simulink model "B2_comparison_tool"  (R2021b)
settings: Solver=VariableStepAuto  StartTime=0.0  StopTime=10  RelTol=1e-3
values from neighbouring files (symbols this model uses):
  K_act = 50    [A10_simple_plant.m]    (also in A11_setup_script_pprz.m = 20; A1_setup_script.m = 20)
  K_act_inner = K_act*eye(4)    [A11_setup_script_pprz.m]    (also in A1_setup_script.m)
  K_ec_u = 1.5    [A11_setup_script_pprz.m]    (also in A1_setup_script.m = 5)
  K_ec_v = 1.5    [A11_setup_script_pprz.m]    (also in A1_setup_script.m = 5)
  K_ec_w = 1.5    [A11_setup_script_pprz.m]    (also in A1_setup_script.m = 5)
  K_u_d = 2.5    [A11_setup_script_pprz.m]    (also in A1_setup_script.m = 7)
  K_v_d = 2.5    [A11_setup_script_pprz.m]    (also in A1_setup_script.m = 7)
  K_w_d = 2.5    [A11_setup_script_pprz.m]    (also in A1_setup_script.m = 7)
  max_motor_rate = 30000    [A11_setup_script_pprz.m]    (also in A1_setup_script.m)
  max_omega_motor = 11000    [A11_setup_script_pprz.m]    (also in A1_setup_script.m)
  omega_c_motors = 50    [A11_setup_script_pprz.m]    (also in A1_setup_script.m)
  sampling_time = 1/frequency    (= 0.002)    [A11_setup_script_pprz.m]    (also in A12_sim_multi_run.m; A1_setup_script.m; A6_slow_actuator.m)
undefined symbols (not defined in the file or in its folder): K_ec_d_p, K_ec_d_q, K_ec_d_r, K_ec_dd_p, K_ec_dd_q, K_ec_dd_r, K_ec_p, K_ec_q, K_ec_r, K_p, K_p_d, K_p_dd, K_q, K_q_d, K_q_dd, K_r, K_r_d, K_r_dd
libraries: dspinverses x16, simulink_extras x8, aerolibutil x2, sharedutil x2, aerolibbdyn x2, aerolibatmos2 x2
(part 2 of 5)

== system B2_comparison_tool/System 0 - New/INDI w// RSPI ==
  " " : Constant  Value=[0;0;0;0]
  Constant : Constant  Value=0
  Constant1 : Constant  Value=max_omega_motor
  Constant2 : Constant  Value=max_motor_rate
  Constant3 : Constant  Value=sampling_time
  Constant4 : Constant  Value=2
  Constant5 : Constant  Value=0
  Demux : Demux
  Demux1 : Demux  Outputs=3
  Demux2 : Demux  Outputs=3
  ERROR CONTROLLER ATTITUDE : Subsystem
  ERROR CONTROLLER VELOCITY : Subsystem
  INTERNAL REFERENCE MODEL ATTITUDE : Subsystem
  INTERNAL REFERENCE MODEL VELOCITY : Subsystem
  MATLAB Function : MATLAB Function  TreatAsAtomicUnit=on
  Scope : Scope
  Scope1 : Scope
  Scope5 : Scope  NumInputPorts=3
  Scope6 : Scope  NumInputPorts=3
  Sum{9..10,14..17} (6 alike) : Sum  Inputs=|+-
  Sum{4..6,11..13} (6 alike) : Sum  Inputs=|++
  Vector Concatenate : Concatenate  NumInputs=6
  pqr_ref : Scope  NumInputPorts=3
  uvw_ref : Scope  NumInputPorts=3
  Motor_1_omega_input : Outport
  Motor_2_omega_input : Outport  Port=2
  Motor_3_omega_input : Outport  Port=3
  Motor_4_omega_input : Outport  Port=4
  wires:
  [Ixx] -> MATLAB Function/1(Ixx)
  [Iyy] -> MATLAB Function/2(Iyy)
  [Izz] -> MATLAB Function/3(Izz)
  [K_m] -> MATLAB Function/4(K_m)
  [K_t] -> MATLAB Function/5(K_t)
  [omega_1] -> MATLAB Function/6(Omega_1)
  [omega_2] -> MATLAB Function/7(Omega_2)
  [omega_3] -> MATLAB Function/8(Omega_3)
  [omega_4] -> MATLAB Function/9(Omega_4)
  [Phi] -> MATLAB Function/10(Phi)
  [Psi] -> MATLAB Function/11(Psi)
  [Theta] -> MATLAB Function/12(Theta)
  [m] -> MATLAB Function/15(m)
  Demux/1 -> Motor_1_omega_input/1
  Demux/2 -> Motor_2_omega_input/1
  Demux/3 -> Motor_3_omega_input/1
  Demux/4 -> Motor_4_omega_input/1
  [dv] -> MATLAB Function/16(dv)
  " "/1 -> MATLAB Function/17(desired_u)
  Constant1/1 -> MATLAB Function/18(max_omega_motor)
  Constant2/1 -> MATLAB Function/19(max_motor_rate)
  Constant3/1 -> MATLAB Function/20(sampling_time)
  MATLAB Function/1(u_out) -> Scope/1, Demux/1
  Constant4/1 -> MATLAB Function/21(max_iter)
  Constant/1 -> INTERNAL REFERENCE MODEL ATTITUDE/1(phi_cmd)
  Constant5/1 -> INTERNAL REFERENCE MODEL ATTITUDE/2(theta_cmd)
  INTERNAL REFERENCE MODEL VELOCITY/5(v_ref) -> ERROR CONTROLLER VELOCITY/2(v_ref), uvw_ref/2
  INTERNAL REFERENCE MODEL ATTITUDE/6(r_ref) -> ERROR CONTROLLER ATTITUDE/3(r_ref), pqr_ref/3
  Demux1/3 -> Sum14/2
  [u_des] -> INTERNAL REFERENCE MODEL VELOCITY/1(u_cmd)
  Sum9/1 -> Vector Concatenate/1
  ERROR CONTROLLER VELOCITY/1(ud_ec) -> Scope6/1, Sum5/2
  [yaw_des] -> INTERNAL REFERENCE MODEL ATTITUDE/3(psi_cmd)
  Vector Concatenate/1 -> Scope1/1, [dv]
  INTERNAL REFERENCE MODEL ATTITUDE/3(rd_ref) -> Sum13/1
  Demux1/1 -> Sum9/2
  INTERNAL REFERENCE MODEL ATTITUDE/5(q_ref) -> ERROR CONTROLLER ATTITUDE/2(q_ref), pqr_ref/2
  Demux2/3 -> Sum17/2
  Sum16/1 -> Vector Concatenate/5
  [pqr_dot_body] -> Demux1/1
  [AxAyAz_earth] -> Demux2/1
  Sum12/1 -> Sum17/1
  Sum10/1 -> Vector Concatenate/2
  Sum14/1 -> Vector Concatenate/3
  ERROR CONTROLLER ATTITUDE/2(qd_ec) -> Scope5/2, Sum11/2
  Demux2/2 -> Sum16/2
  ERROR CONTROLLER ATTITUDE/1(pd_ec) -> Scope5/1, Sum4/2
  Sum15/1 -> Vector Concatenate/4
  Sum17/1 -> Vector Concatenate/6
  ERROR CONTROLLER VELOCITY/3(wd_ec) -> Scope6/3, Sum12/2
  Sum11/1 -> Sum10/1
  INTERNAL REFERENCE MODEL VELOCITY/4(u_ref) -> uvw_ref/1, ERROR CONTROLLER VELOCITY/1(u_ref)
  Sum13/1 -> Sum14/1
  Sum6/1 -> Sum16/1
  INTERNAL REFERENCE MODEL VELOCITY/6(w_ref) -> ERROR CONTROLLER VELOCITY/3(w_ref), uvw_ref/3
  [v_des] -> INTERNAL REFERENCE MODEL VELOCITY/2(v_cmd)
  Demux1/2 -> Sum10/2
  ERROR CONTROLLER VELOCITY/2(vd_ec) -> Scope6/2, Sum6/2
  INTERNAL REFERENCE MODEL VELOCITY/1(ud_ref) -> Sum5/1
  [w_des] -> INTERNAL REFERENCE MODEL VELOCITY/3(w_cmd)
  Sum5/1 -> Sum15/1
  INTERNAL REFERENCE MODEL VELOCITY/3(wd_ref) -> Sum12/1
  Demux2/1 -> Sum15/2
  INTERNAL REFERENCE MODEL ATTITUDE/7(phi_ref) -> ERROR CONTROLLER ATTITUDE/4(phi_ref)
  INTERNAL REFERENCE MODEL ATTITUDE/8(theta_ref) -> ERROR CONTROLLER ATTITUDE/5(theta_ref)
  INTERNAL REFERENCE MODEL ATTITUDE/1(pd_ref) -> Sum4/1
  INTERNAL REFERENCE MODEL VELOCITY/2(vd_ref) -> Sum6/1
  Sum4/1 -> Sum9/1
  INTERNAL REFERENCE MODEL ATTITUDE/4(p_ref) -> pqr_ref/1, ERROR CONTROLLER ATTITUDE/1(p_ref)
  INTERNAL REFERENCE MODEL ATTITUDE/9(psi_ref) -> ERROR CONTROLLER ATTITUDE/6(psi_ref)
  INTERNAL REFERENCE MODEL ATTITUDE/2(qd_ref) -> Sum11/1
  ERROR CONTROLLER ATTITUDE/3(qr_ec) -> Scope5/3, Sum13/2
  [b] -> MATLAB Function/13(b)
  [l] -> MATLAB Function/14(l)

== system B2_comparison_tool/System 0 - New/Quadcopter Characteristics ==
  Gravity : Constant  Value=9.80665
  Moment Gain : Constant  Value=6.68*10^-10
  Plate Distance from CG : Constant  Value=0.1
  Plate Radius (cm) : Constant  Value=0.30
  Quad Inertia Ixx [kg*m^2] : Constant  Value=0.0012458
  Quad Inertia Iyy [kg*m^2] : Constant  Value=0.001500
  Quad Inertia Izz [kg*m^2] : Constant  Value=0.0001500
  Quad Mass [kg] : Constant  Value=0.4
  Thrust Gain : Constant  Value=6.557*10^-8
  lx1 : Constant  Value=0.095
  lx2 : Constant  Value=0.08
  tag scope: Ixx=global, Iyy=global, Izz=global, K_m=global, K_t=global, b=global, g=global, l=global, l_plate=global, m=global, r_plate=global
  wires:
  Quad Inertia Ixx [kg*m^2]/1 -> [Ixx]
  Quad Inertia Iyy [kg*m^2]/1 -> [Iyy]
  Quad Inertia Izz [kg*m^2]/1 -> [Izz]
  Quad Mass [kg]/1 -> [m]
  Thrust Gain/1 -> [K_t]
  Moment Gain/1 -> [K_m]
  lx1/1 -> [b]
  lx2/1 -> [l]
  Plate Radius (cm)/1 -> [r_plate]
  Plate Distance from CG/1 -> [l_plate]
  Gravity/1 -> [g]

== system B2_comparison_tool/System 1 - Old/Actuator Dynamics Block ==
  Motor_1_omega_input : Inport
  Motor_2_omega_input : Inport  Port=2
  Motor_3_omega_input : Inport  Port=3
  Motor_4_omega_input : Inport  Port=4
  Clock : Clock
  Constant : Constant  Value=.1
  Constant1 : Constant  Value=1000
  Constant2 : Constant  Value=1000
  Display : Display
  Display1 : Display
  Display2 : Display
  Saturation{1..4} (4 alike) : Saturate  UpperLimit=max_omega_motor  LowerLimit=10
  Scope : Scope  NumInputPorts=4
  Sum : Sum  Inputs=|+-
  Switch{,1..3} (4 alike) : Switch  Criteria=u2 > Threshold
  Transfer Fcn{,1..3} (4 alike) : TransferFcn  Numerator=[omega_c_motors]  Denominator=[1 omega_c_motors]
  omega_1 : Outport
  omega_2 : Outport  Port=2
  omega_3 : Outport  Port=3
  omega_4 : Outport  Port=4
  wires:
  Sum/1 -> Switch3/2, Switch2/2, Switch1/2, Switch/2
  Constant1/1 -> Switch/3, Switch1/3
  Switch1/1 -> Scope/2, omega_2/1
  Transfer Fcn2/1 -> Switch2/1  "omega_3"
  Constant/1 -> Sum/2
  Motor_3_omega_input/1 -> Saturation2/1  "omega_3_in"
  Constant2/1 -> Switch2/3, Switch3/3
  Switch3/1 -> Scope/4, omega_4/1
  Transfer Fcn/1 -> Display1/1, Switch/1  "omega_1"
  Motor_4_omega_input/1 -> Saturation3/1  "omega_4_in"
  Saturation1/1 -> Transfer Fcn1/1
  Transfer Fcn3/1 -> Switch3/1  "omega_4"
  Switch/1 -> Display2/1, Scope/1, omega_1/1
  Saturation2/1 -> Transfer Fcn2/1
  Saturation3/1 -> Transfer Fcn3/1
  Saturation4/1 -> Transfer Fcn/1
  Transfer Fcn1/1 -> Switch1/1  "omega_2"
  Motor_2_omega_input/1 -> Saturation1/1  "omega_2_in"
  Motor_1_omega_input/1 -> Display/1, Saturation4/1  "omega_1_in"
  Clock/1 -> Sum/1
  Switch2/1 -> Scope/3, omega_3/1

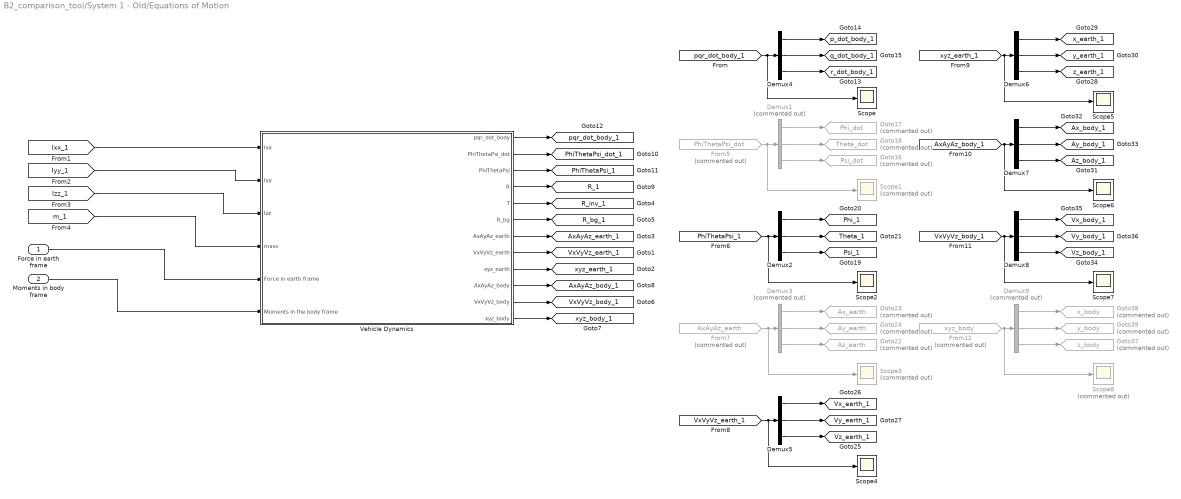
== system B2_comparison_tool/System 1 - Old/Equations of Motion ==
  Force in earth frame : Inport
  Moments in body frame : Inport  Port=2
  Demux1 : Demux  Commented=on  Outputs=3
  Demux{2,4..8} (6 alike) : Demux  Outputs=3
  Demux3 : Demux  Commented=on  Outputs=3
  Demux9 : Demux  Commented=on  Outputs=3
  From12 : From  Commented=on  GotoTag=xyz_body  TagVisibility=global
  From5 : From  Commented=on  GotoTag=PhiThetaPsi_dot  TagVisibility=global
  From7 : From  Commented=on  GotoTag=AxAyAz_earth  TagVisibility=global
  Goto16 : Goto  Commented=on  GotoTag=Psi_dot  TagVisibility=global
  Goto17 : Goto  Commented=on  GotoTag=Phi_dot  TagVisibility=global
  Goto18 : Goto  Commented=on  GotoTag=Theta_dot  TagVisibility=global
  Goto22 : Goto  Commented=on  GotoTag=Az_earth  TagVisibility=global
  Goto23 : Goto  Commented=on  GotoTag=Ax_earth  TagVisibility=global
  Goto24 : Goto  Commented=on  GotoTag=Ay_earth  TagVisibility=global
  Goto37 : Goto  Commented=on  GotoTag=z_body  TagVisibility=global
  Goto38 : Goto  Commented=on  GotoTag=x_body  TagVisibility=global
  Goto39 : Goto  Commented=on  GotoTag=y_body  TagVisibility=global
  Scope{,2,4..7} (6 alike) : Scope
  Scope1 : Scope  Commented=on
  Scope3 : Scope  Commented=on
  Scope8 : Scope  Commented=on
  Vehicle Dynamics : Subsystem
  tag scope: AxAyAz_body_1=global, AxAyAz_earth_1=global, Ax_body_1=global, Ay_body_1=global, Az_body_1=global, PhiThetaPsi_1=global, PhiThetaPsi_dot_1=global, Phi_1=global, Psi_1=global, R_1=global, R_bg_1=global, R_inv_1=global, Theta_1=global, VxVyVz_body_1=global, VxVyVz_earth_1=global, Vx_body_1=global, Vx_earth_1=global, Vy_body_1=global, Vy_earth_1=global, Vz_body_1=global, Vz_earth_1=global, p_dot_body_1=global, pqr_dot_body_1=global, q_dot_body_1=global, r_dot_body_1=global, x_earth_1=global, xyz_body_1=global, xyz_earth_1=global, y_earth_1=global, z_earth_1=global
  wires:
  Force in earth frame/1 -> Vehicle Dynamics/5(Force in earth frame)
  Moments in body frame/1 -> Vehicle Dynamics/6(Moments in the body frame)
  [m_1] -> Vehicle Dynamics/4(mass)
  [Izz_1] -> Vehicle Dynamics/3(Izz)
  [Iyy_1] -> Vehicle Dynamics/2(Iyy)
  [Ixx_1] -> Vehicle Dynamics/1(Ixx)
  Vehicle Dynamics/5(T) -> [R_inv_1]
  Vehicle Dynamics/4(R) -> [R_1]
  Vehicle Dynamics/6(R_bg) -> [R_bg_1]
  Vehicle Dynamics/1(pqr_dot_body) -> [pqr_dot_body_1]
  Vehicle Dynamics/2(PhiThetaPsi_dot) -> [PhiThetaPsi_dot_1]
  Vehicle Dynamics/3(PhiThetaPsi) -> [PhiThetaPsi_1]
  Vehicle Dynamics/7(AxAyAz_earth) -> [AxAyAz_earth_1]
  Vehicle Dynamics/8(VxVyVz_earth) -> [VxVyVz_earth_1]
  Vehicle Dynamics/9(xyz_earth) -> [xyz_earth_1]
  Vehicle Dynamics/10(AxAyAz_body) -> [AxAyAz_body_1]
  Vehicle Dynamics/11(VxVyVz_body) -> [VxVyVz_body_1]
  Vehicle Dynamics/12(xyz_body) -> [xyz_body_1]
  From12/1 -> Scope8/1, Demux9/1
  Demux4/1 -> [p_dot_body_1]
  [xyz_earth_1] -> Scope5/1, Demux6/1
  From5/1 -> Scope1/1, Demux1/1
  Demux7/1 -> [Ax_body_1]
  [PhiThetaPsi_1] -> Scope2/1, Demux2/1
  Demux7/2 -> [Ay_body_1]
  Demux6/3 -> [z_earth_1]
  Demux8/1 -> [Vx_body_1]
  Demux9/3 -> Goto37/1
  Demux9/2 -> Goto39/1
  Demux1/2 -> Goto18/1
  Demux3/1 -> Goto23/1
  Demux8/3 -> [Vz_body_1]
  [VxVyVz_body_1] -> Scope7/1, Demux8/1
  Demux8/2 -> [Vy_body_1]
  From7/1 -> Scope3/1, Demux3/1
  Demux3/2 -> Goto24/1
  Demux7/3 -> [Az_body_1]
  [AxAyAz_body_1] -> Scope6/1, Demux7/1
  Demux5/1 -> [Vx_earth_1]
  Demux1/1 -> Goto17/1
  Demux2/1 -> [Phi_1]
  [VxVyVz_earth_1] -> Scope4/1, Demux5/1
  Demux5/2 -> [Vy_earth_1]
  Demux9/1 -> Goto38/1
  Demux5/3 -> [Vz_earth_1]
  Demux2/3 -> [Psi_1]
  Demux1/3 -> Goto16/1
  Demux6/2 -> [y_earth_1]
  Demux3/3 -> Goto22/1
  Demux2/2 -> [Theta_1]
  Demux4/3 -> [r_dot_body_1]
  [pqr_dot_body_1] -> Scope/1, Demux4/1
  Demux6/1 -> [x_earth_1]
  Demux4/2 -> [q_dot_body_1]

== system B2_comparison_tool/System 1 - Old/Force and Moment Calculation ==
  omega_1 : Inport
  omega_2 : Inport  Port=2
  omega_3 : Inport  Port=3
  omega_4 : Inport  Port=4
  Add : Sum
  Add1 : Sum
  Demux : Demux  Outputs=3
  Demux1 : Demux  Outputs=3
  Forces : Scope  NumInputPorts=3
  Forces and Moments due to Aerodynamic Forces : Subsystem
  Forces due to thrust : MATLAB Function  TreatAsAtomicUnit=on
  Moments : Scope  NumInputPorts=3
  Moments due to thrust : MATLAB Function  TreatAsAtomicUnit=on
  Scope : Scope
  Force in the earth frame : Outport
  Moments in body frame : Outport  Port=2
  tag scope: Fx_earth_1=global, Fy_earth_2=global, Fz_earth_3=global, Mx_1=global, My_1=global, Mz_1=global, T_1=global, omega_1_1=global, omega_2_1=global, omega_3_1=global, omega_4_1=global
  wires:
  omega_1/1 -> [omega_1_1]
  omega_4/1 -> [omega_4_1]
  omega_3/1 -> [omega_3_1]
  omega_2/1 -> [omega_2_1]
  [omega_4_1] -> Forces due to thrust/4(omega_4)
  [omega_3_1] -> Forces due to thrust/3(omega_3)
  [omega_2_1] -> Forces due to thrust/2(omega_2)
  [omega_1_1] -> Forces due to thrust/1(omega_1)
  [R_bg_1] -> Forces due to thrust/5(R_bg)
  [K_t_1] -> Forces due to thrust/6(K_t)
  Forces due to thrust/1(F_t_e) -> Forces/2, Add/2  "thrust_force"
  Add/1 -> Forces/3, Force in the earth frame/1, Demux/1  "total_force"
  [R_bg_1] -> Forces and Moments due to Aerodynamic Forces/2(R_bg)
  [z_earth_1] -> Forces and Moments due to Aerodynamic Forces/1(z_earth)
  Forces and Moments due to Aerodynamic Forces/1(F_aero) -> Add/1, Forces/1  "aero_force"
  Moments due to thrust/1(M_t) -> Moments/2, Add1/2, Scope/1  "thrust_moment"
  [omega_1_1] -> Moments due to thrust/1(omega_1)
  [omega_2_1] -> Moments due to thrust/2(omega_2)
  [omega_3_1] -> Moments due to thrust/3(omega_3)
  [omega_4_1] -> Moments due to thrust/4(omega_4)
  [K_t_1] -> Moments due to thrust/5(K_t)
  [K_m_1] -> Moments due to thrust/6(K_m)
  Add1/1 -> Moments/3, Moments in body frame/1, Demux1/1  "full_moment"
  Demux/1 -> [Fx_earth_1]
  Demux/3 -> [Fz_earth_3]
  Demux/2 -> [Fy_earth_2]
  Demux1/2 -> [My_1]
  Demux1/1 -> [Mx_1]
  Demux1/3 -> [Mz_1]
  Forces due to thrust/2(F_t_b) -> [T_1]
  [b_1] -> Moments due to thrust/7(b)
  [l_1] -> Moments due to thrust/8(l)
  Forces and Moments due to Aerodynamic Forces/2(M_aero) -> Add1/1, Moments/1  "aero_moment"

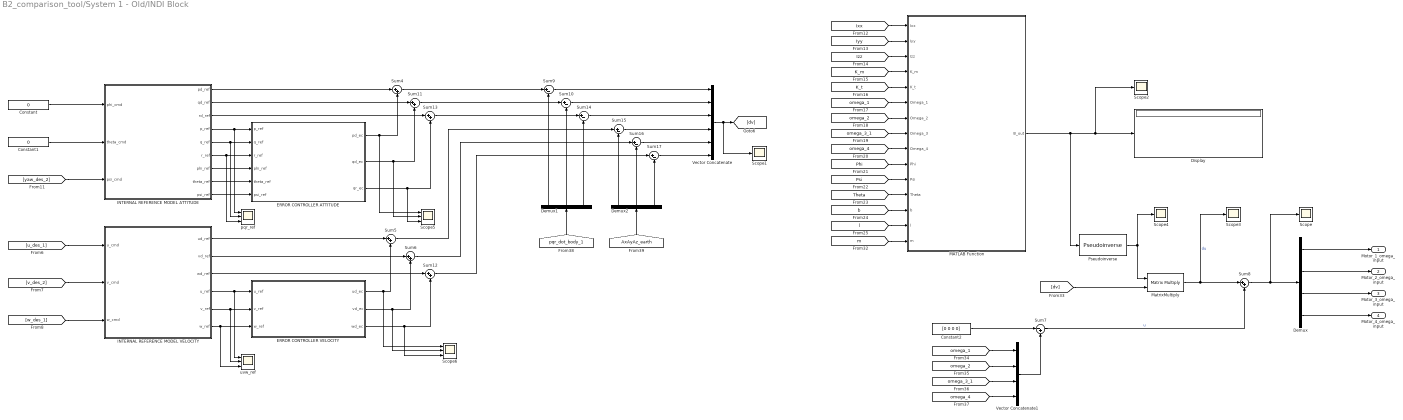
== system B2_comparison_tool/System 1 - Old/INDI Block ==
  Constant : Constant  Value=0
  Constant1 : Constant  Value=0
  Constant2 : Constant  Value=[0 0 0 0]
  Demux : Demux
  Demux1 : Demux  Outputs=3
  Demux2 : Demux  Outputs=3
  Display : Display
  ERROR CONTROLLER ATTITUDE : Subsystem
  ERROR CONTROLLER VELOCITY : Subsystem
  INTERNAL REFERENCE MODEL ATTITUDE : Subsystem
  INTERNAL REFERENCE MODEL VELOCITY : Subsystem
  MATLAB Function : MATLAB Function  TreatAsAtomicUnit=on
  MatrixMultiply : Product  Multiplication=Matrix(*)
  Pseudoinverse : dspinverses/Pseudoinverse  wanterr=off  SimulateUsing=Interpreted execution
      settings: SourceProductBaseCode=DS
  Scope{,1..4} (5 alike) : Scope
  Scope5 : Scope  NumInputPorts=3
  Scope6 : Scope  NumInputPorts=3
  Sum{9..10,14..17} (6 alike) : Sum  Inputs=|+-
  Sum{4..6,8,11..13} (7 alike) : Sum  Inputs=|++
  Sum7 : Sum  Inputs=|-+
  Vector Concatenate : Concatenate  NumInputs=6
  Vector Concatenate1 : Concatenate  NumInputs=4
  pqr_ref : Scope  NumInputPorts=3
  uvw_ref : Scope  NumInputPorts=3
  Motor_1_omega_input : Outport
  Motor_2_omega_input : Outport  Port=2
  Motor_3_omega_input : Outport  Port=3
  Motor_4_omega_input : Outport  Port=4
  wires:
  ERROR CONTROLLER ATTITUDE/2(qd_ec) -> Scope5/2, Sum11/2
  INTERNAL REFERENCE MODEL ATTITUDE/2(qd_ref) -> Sum11/1
  INTERNAL REFERENCE MODEL ATTITUDE/1(pd_ref) -> Sum4/1
  INTERNAL REFERENCE MODEL ATTITUDE/5(q_ref) -> ERROR CONTROLLER ATTITUDE/2(q_ref), pqr_ref/2
  INTERNAL REFERENCE MODEL ATTITUDE/9(psi_ref) -> ERROR CONTROLLER ATTITUDE/6(psi_ref)
  INTERNAL REFERENCE MODEL ATTITUDE/6(r_ref) -> ERROR CONTROLLER ATTITUDE/3(r_ref), pqr_ref/3
  INTERNAL REFERENCE MODEL ATTITUDE/4(p_ref) -> pqr_ref/1, ERROR CONTROLLER ATTITUDE/1(p_ref)
  INTERNAL REFERENCE MODEL ATTITUDE/3(rd_ref) -> Sum13/1
  ERROR CONTROLLER ATTITUDE/3(qr_ec) -> Scope5/3, Sum13/2
  INTERNAL REFERENCE MODEL ATTITUDE/7(phi_ref) -> ERROR CONTROLLER ATTITUDE/4(phi_ref)
  ERROR CONTROLLER ATTITUDE/1(pd_ec) -> Scope5/1, Sum4/2
  INTERNAL REFERENCE MODEL ATTITUDE/8(theta_ref) -> ERROR CONTROLLER ATTITUDE/5(theta_ref)
  ERROR CONTROLLER VELOCITY/1(ud_ec) -> Scope6/1, Sum5/2
  ERROR CONTROLLER VELOCITY/3(wd_ec) -> Scope6/3, Sum12/2
  INTERNAL REFERENCE MODEL VELOCITY/3(wd_ref) -> Sum12/1
  INTERNAL REFERENCE MODEL VELOCITY/2(vd_ref) -> Sum6/1
  INTERNAL REFERENCE MODEL VELOCITY/5(v_ref) -> ERROR CONTROLLER VELOCITY/2(v_ref), uvw_ref/2
  Sum12/1 -> Sum17/1
  INTERNAL REFERENCE MODEL VELOCITY/6(w_ref) -> ERROR CONTROLLER VELOCITY/3(w_ref), uvw_ref/3
  Sum5/1 -> Sum15/1
  INTERNAL REFERENCE MODEL VELOCITY/1(ud_ref) -> Sum5/1
  ERROR CONTROLLER VELOCITY/2(vd_ec) -> Scope6/2, Sum6/2
  INTERNAL REFERENCE MODEL VELOCITY/4(u_ref) -> uvw_ref/1, ERROR CONTROLLER VELOCITY/1(u_ref)
  Sum6/1 -> Sum16/1
  [u_des_1] -> INTERNAL REFERENCE MODEL VELOCITY/1(u_cmd)
  [v_des_2] -> INTERNAL REFERENCE MODEL VELOCITY/2(v_cmd)
  [w_des_1] -> INTERNAL REFERENCE MODEL VELOCITY/3(w_cmd)
  Constant/1 -> INTERNAL REFERENCE MODEL ATTITUDE/1(phi_cmd)
  Constant1/1 -> INTERNAL REFERENCE MODEL ATTITUDE/2(theta_cmd)
  [yaw_des_2] -> INTERNAL REFERENCE MODEL ATTITUDE/3(psi_cmd)
  Sum4/1 -> Sum9/1
  Sum11/1 -> Sum10/1
  Sum13/1 -> Sum14/1
  Vector Concatenate/1 -> Scope1/1, [dv]
  [Ixx] -> MATLAB Function/1(Ixx)
  [Iyy] -> MATLAB Function/2(Iyy)
  [Izz] -> MATLAB Function/3(Izz)
  [K_m] -> MATLAB Function/4(K_m)
  [K_t] -> MATLAB Function/5(K_t)
  [omega_1] -> MATLAB Function/6(Omega_1)
  [omega_2] -> MATLAB Function/7(Omega_2)
  [omega_3_1] -> MATLAB Function/8(Omega_3)
  [omega_4] -> MATLAB Function/9(Omega_4)
  [Phi] -> MATLAB Function/10(Phi)
  [Psi] -> MATLAB Function/11(Psi)
  [Theta] -> MATLAB Function/12(Theta)
  [b] -> MATLAB Function/13(b)
  [l] -> MATLAB Function/14(l)
  [m] -> MATLAB Function/15(m)
  MATLAB Function/1(B_out) -> Pseudoinverse/1, Scope2/1, Display/1
  Pseudoinverse/1 -> MatrixMultiply/1, Scope4/1
  MatrixMultiply/1 -> Scope3/1, Sum8/1  "du"
  [omega_1] -> Vector Concatenate1/1
  [omega_2] -> Vector Concatenate1/2
  [omega_3_1] -> Vector Concatenate1/3
  [omega_4] -> Vector Concatenate1/4
  Vector Concatenate1/1 -> Sum7/2
  Constant2/1 -> Sum7/1
  Sum7/1 -> Sum8/2  "u"
  Sum8/1 -> Scope/1, Demux/1
  Demux/1 -> Motor_1_omega_input/1
  Demux/2 -> Motor_2_omega_input/1
  Demux/3 -> Motor_3_omega_input/1
  Demux/4 -> Motor_4_omega_input/1
  Sum9/1 -> Vector Concatenate/1
  Sum10/1 -> Vector Concatenate/2
  Sum14/1 -> Vector Concatenate/3
  Sum15/1 -> Vector Concatenate/4
  Sum16/1 -> Vector Concatenate/5
  Sum17/1 -> Vector Concatenate/6
  [pqr_dot_body_1] -> Demux1/1
  [AxAyAz_earth] -> Demux2/1
  Demux2/3 -> Sum17/2
  Demux2/2 -> Sum16/2
  Demux2/1 -> Sum15/2
  Demux1/3 -> Sum14/2
  Demux1/2 -> Sum10/2
  Demux1/1 -> Sum9/2
  [dv] -> MatrixMultiply/2

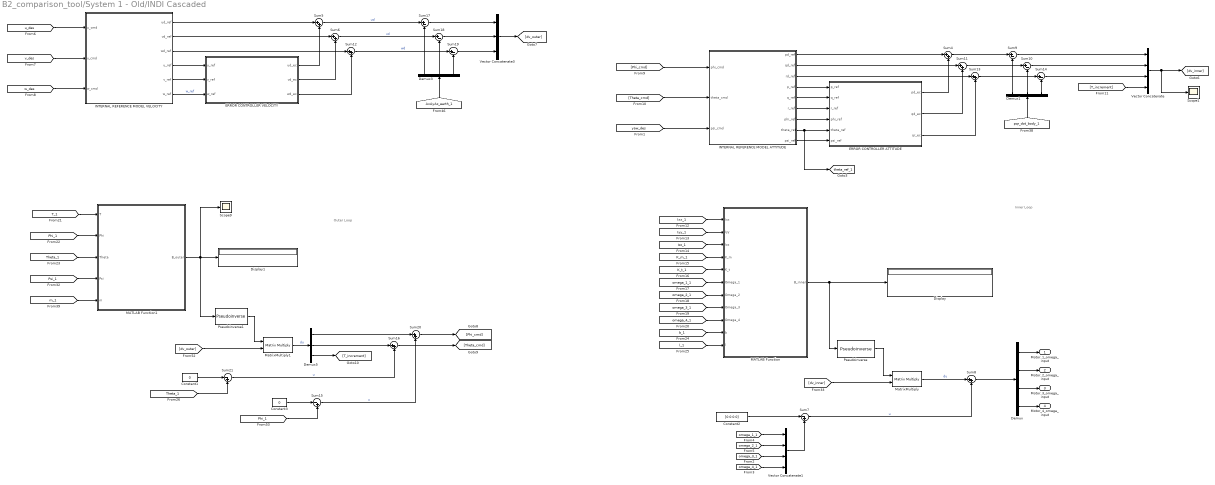
== system B2_comparison_tool/System 1 - Old/INDI Cascaded ==
  note: Outer Loop
  note: Inner Loop
  Constant1 : Constant  Value=0
  Constant2 : Constant  Value=[0 0 0 0]
  Constant3 : Constant  Value=0
  Demux : Demux
  Demux1 : Demux  Outputs=3
  Demux3 : Demux  Outputs=3
  Demux5 : Demux  Outputs=3
  Display : Display
  Display1 : Display
  ERROR CONTROLLER ATTITUDE : Subsystem
  ERROR CONTROLLER VELOCITY : Subsystem
  INTERNAL REFERENCE MODEL ATTITUDE : Subsystem
  INTERNAL REFERENCE MODEL VELOCITY : Subsystem
  MATLAB Function : MATLAB Function  TreatAsAtomicUnit=on
  MATLAB Function1 : MATLAB Function  TreatAsAtomicUnit=on
  MatrixMultiply : Product  Multiplication=Matrix(*)
  MatrixMultiply1 : Product  Multiplication=Matrix(*)
  Pseudoinverse : dspinverses/Pseudoinverse  wanterr=off  SimulateUsing=Interpreted execution
      settings: SourceProductBaseCode=DS
  Pseudoinverse1 : dspinverses/Pseudoinverse  wanterr=off  SimulateUsing=Interpreted execution
      settings: SourceProductBaseCode=DS
  Scope1 : Scope
  Scope9 : Scope
  Sum{9..10,14,17..19} (6 alike) : Sum  Inputs=|+-
  Sum{4..6,8,11..13,16,20} (9 alike) : Sum  Inputs=|++
  Sum15 : Sum  Inputs=|-+
  Sum21 : Sum  Inputs=|-+
  Sum7 : Sum  Inputs=|-+
  Vector Concatenate : Concatenate  NumInputs=4
  Vector Concatenate1 : Concatenate  NumInputs=4
  Vector Concatenate3 : Concatenate  NumInputs=3
  Motor_1_omega_input : Outport
  Motor_2_omega_input : Outport  Port=2
  Motor_3_omega_input : Outport  Port=3
  Motor_4_omega_input : Outport  Port=4
  tag scope: theta_ref_1=global
  wires:
  ERROR CONTROLLER ATTITUDE/2(qd_ec) -> Sum11/2
  INTERNAL REFERENCE MODEL ATTITUDE/2(qd_ref) -> Sum11/1
  INTERNAL REFERENCE MODEL ATTITUDE/1(pd_ref) -> Sum4/1
  INTERNAL REFERENCE MODEL ATTITUDE/5(q_ref) -> ERROR CONTROLLER ATTITUDE/2(q_ref)
  INTERNAL REFERENCE MODEL ATTITUDE/9(psi_ref) -> ERROR CONTROLLER ATTITUDE/6(psi_ref)
  INTERNAL REFERENCE MODEL ATTITUDE/6(r_ref) -> ERROR CONTROLLER ATTITUDE/3(r_ref)
  INTERNAL REFERENCE MODEL ATTITUDE/4(p_ref) -> ERROR CONTROLLER ATTITUDE/1(p_ref)
  INTERNAL REFERENCE MODEL ATTITUDE/3(rd_ref) -> Sum13/1
  ERROR CONTROLLER ATTITUDE/3(qr_ec) -> Sum13/2
  INTERNAL REFERENCE MODEL ATTITUDE/7(phi_ref) -> ERROR CONTROLLER ATTITUDE/4(phi_ref)
  ERROR CONTROLLER ATTITUDE/1(pd_ec) -> Sum4/2
  INTERNAL REFERENCE MODEL ATTITUDE/8(theta_ref) -> [theta_ref_1], ERROR CONTROLLER ATTITUDE/5(theta_ref)
  ERROR CONTROLLER VELOCITY/1(ud_ec) -> Sum5/2
  ERROR CONTROLLER VELOCITY/3(wd_ec) -> Sum12/2
  INTERNAL REFERENCE MODEL VELOCITY/3(wd_ref) -> Sum12/1
  INTERNAL REFERENCE MODEL VELOCITY/2(vd_ref) -> Sum6/1
  INTERNAL REFERENCE MODEL VELOCITY/5(v_ref) -> ERROR CONTROLLER VELOCITY/2(v_ref)
  INTERNAL REFERENCE MODEL VELOCITY/6(w_ref) -> ERROR CONTROLLER VELOCITY/3(w_ref)  "w_ref"
  INTERNAL REFERENCE MODEL VELOCITY/1(ud_ref) -> Sum5/1
  ERROR CONTROLLER VELOCITY/2(vd_ec) -> Sum6/2
  INTERNAL REFERENCE MODEL VELOCITY/4(u_ref) -> ERROR CONTROLLER VELOCITY/1(u_ref)
  [u_des] -> INTERNAL REFERENCE MODEL VELOCITY/1(u_cmd)
  [v_des] -> INTERNAL REFERENCE MODEL VELOCITY/2(v_cmd)
  [w_des] -> INTERNAL REFERENCE MODEL VELOCITY/3(w_cmd)
  [Phi_cmd] -> INTERNAL REFERENCE MODEL ATTITUDE/1(phi_cmd)
  [Theta_cmd] -> INTERNAL REFERENCE MODEL ATTITUDE/2(theta_cmd)
  [yaw_des] -> INTERNAL REFERENCE MODEL ATTITUDE/3(psi_cmd)
  Vector Concatenate/1 -> Scope1/1, [dv_inner]
  MATLAB Function/1(B_inner) -> Pseudoinverse/1, Display/1
  Pseudoinverse/1 -> MatrixMultiply/1
  MatrixMultiply/1 -> Sum8/1  "du"
  [omega_1_1] -> Vector Concatenate1/1
  [omega_2_1] -> Vector Concatenate1/2
  [omega_3_1] -> Vector Concatenate1/3
  [omega_4_1] -> Vector Concatenate1/4
  Vector Concatenate1/1 -> Sum7/2
  Constant2/1 -> Sum7/1
  Sum7/1 -> Sum8/2  "u"
  Sum8/1 -> Demux/1
  Demux/1 -> Motor_1_omega_input/1
  Demux/2 -> Motor_2_omega_input/1
  Demux/3 -> Motor_3_omega_input/1
  Demux/4 -> Motor_4_omega_input/1
  Sum9/1 -> Vector Concatenate/1
  Sum10/1 -> Vector Concatenate/2
  Sum14/1 -> Vector Concatenate/3
  [pqr_dot_body_1] -> Demux1/1
  Demux1/3 -> Sum14/2
  Demux1/2 -> Sum10/2
  Demux1/1 -> Sum9/2
  [dv_inner] -> MatrixMultiply/2
  [T_increment] -> Vector Concatenate/4
  Sum4/1 -> Sum9/1
  Sum11/1 -> Sum10/1
  Sum13/1 -> Sum14/1
  Sum12/1 -> Sum19/1  "wd"
  Sum6/1 -> Sum18/1  "vd"
  Sum5/1 -> Sum17/1  "ud"
  Vector Concatenate3/1 -> [dv_outer]
  Sum19/1 -> Vector Concatenate3/3
  Sum18/1 -> Vector Concatenate3/2
  Sum17/1 -> Vector Concatenate3/1
  [AxAyAz_earth_1] -> Demux3/1
  Demux3/3 -> Sum19/2
  Demux3/2 -> Sum18/2
  Demux3/1 -> Sum17/2
  [K_m_1] -> MATLAB Function/4(K_m)
  [Izz_1] -> MATLAB Function/3(Izz)
  [Iyy_1] -> MATLAB Function/2(Iyy)
  [Ixx_1] -> MATLAB Function/1(Ixx)
  [omega_3_1] -> MATLAB Function/8(Omega_3)
  [omega_1_1] -> MATLAB Function/6(Omega_1)
  [omega_4_1] -> MATLAB Function/9(Omega_4)
  [K_t_1] -> MATLAB Function/5(K_t)
  [b_1] -> MATLAB Function/10(b)
  [l_1] -> MATLAB Function/11(l)
  [omega_2_1] -> MATLAB Function/7(Omega_2)
  Pseudoinverse1/1 -> MatrixMultiply1/1
  Sum20/1 -> [Phi_cmd]
  Demux5/1 -> Sum20/1
  [Phi_1] -> MATLAB Function1/2(Phi)
  Demux5/2 -> Sum16/1
  MatrixMultiply1/1 -> Demux5/1  "du"
  Sum21/1 -> Sum16/2  "u"
  [Theta_1] -> Sum21/2
  [m_1] -> MATLAB Function1/5(m)
  [T_1] -> MATLAB Function1/1(T)
  [dv_outer] -> MatrixMultiply1/2
  Constant1/1 -> Sum21/1
  [Phi_1] -> Sum15/2
  Sum16/1 -> [Theta_cmd]
  [Psi_1] -> MATLAB Function1/4(Psi)
  [Theta_1] -> MATLAB Function1/3(Theta)
  Demux5/3 -> [T_increment]
  Sum15/1 -> Sum20/2  "u"
  MATLAB Function1/1(B_outer) -> Pseudoinverse1/1, Scope9/1, Display1/1
  Constant3/1 -> Sum15/1

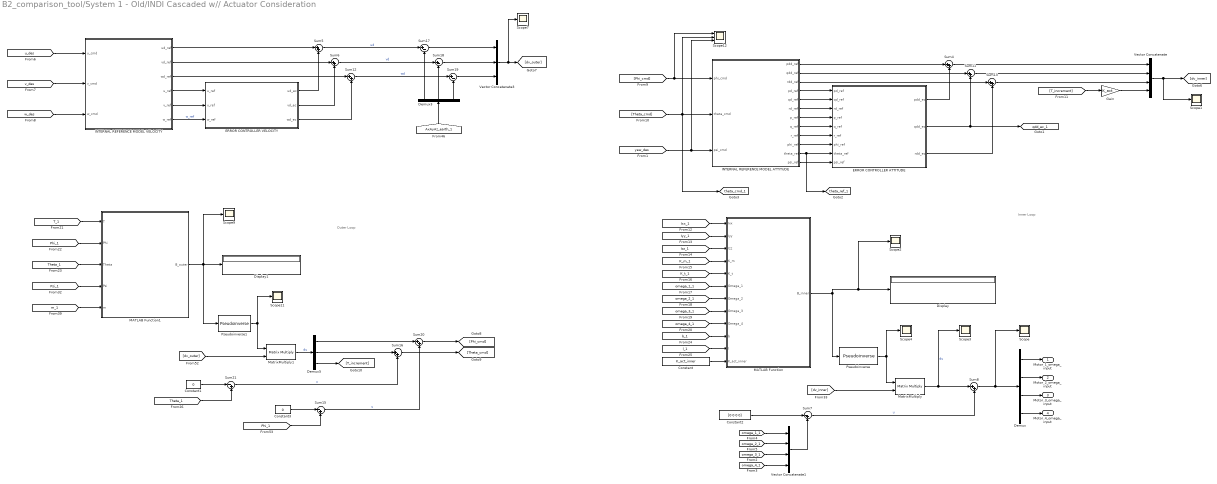
== system B2_comparison_tool/System 1 - Old/INDI Cascaded w// Actuator Consideration ==
  note: Outer Loop
  note: Inner Loop
  Constant : Constant  Value=K_act_inner
  Constant1 : Constant  Value=0
  Constant2 : Constant  Value=[0 0 0 0]
  Constant3 : Constant  Value=0
  Demux : Demux
  Demux3 : Demux  Outputs=3
  Demux5 : Demux  Outputs=3
  Display : Display
  Display1 : Display
  ERROR CONTROLLER ATTITUDE : Subsystem
  ERROR CONTROLLER VELOCITY : Subsystem
  Gain : Gain  Gain=K_act
  INTERNAL REFERENCE MODEL ATTITUDE : Subsystem
  INTERNAL REFERENCE MODEL VELOCITY : Subsystem
  MATLAB Function : MATLAB Function  TreatAsAtomicUnit=on
  MATLAB Function1 : MATLAB Function  TreatAsAtomicUnit=on
  MatrixMultiply : Product  Multiplication=Matrix(*)
  MatrixMultiply1 : Product  Multiplication=Matrix(*)
  Pseudoinverse : dspinverses/Pseudoinverse  wanterr=off  SimulateUsing=Interpreted execution
      settings: SourceProductBaseCode=DS
  Pseudoinverse1 : dspinverses/Pseudoinverse  wanterr=off  SimulateUsing=Interpreted execution
      settings: SourceProductBaseCode=DS
  Scope{,1..4,7,9,11} (8 alike) : Scope
  Scope12 : Scope  NumInputPorts=3
  Sum{4..6,8,11..13,16,20} (9 alike) : Sum  Inputs=|++
  Sum15 : Sum  Inputs=|-+
  Sum17 : Sum  Inputs=|+-
  Sum18 : Sum  Inputs=|+-
  Sum19 : Sum  Inputs=|+-
  Sum21 : Sum  Inputs=|-+
  Sum7 : Sum  Inputs=|-+
  Vector Concatenate : Concatenate  NumInputs=4
  Vector Concatenate1 : Concatenate  NumInputs=4
  Vector Concatenate3 : Concatenate  NumInputs=3
  Motor_1_omega_input : Outport
  Motor_2_omega_input : Outport  Port=2
  Motor_3_omega_input : Outport  Port=3
  Motor_4_omega_input : Outport  Port=4
  tag scope: qdd_ec_1=global, theta_cmd_1=global, theta_ref_1=global
  wires:
  ERROR CONTROLLER VELOCITY/1(ud_ec) -> Sum5/2
  ERROR CONTROLLER VELOCITY/3(wd_ec) -> Sum12/2
  INTERNAL REFERENCE MODEL VELOCITY/3(wd_ref) -> Sum12/1
  INTERNAL REFERENCE MODEL VELOCITY/2(vd_ref) -> Sum6/1
  INTERNAL REFERENCE MODEL VELOCITY/5(v_ref) -> ERROR CONTROLLER VELOCITY/2(v_ref)
  INTERNAL REFERENCE MODEL VELOCITY/6(w_ref) -> ERROR CONTROLLER VELOCITY/3(w_ref)  "w_ref"
  INTERNAL REFERENCE MODEL VELOCITY/1(ud_ref) -> Sum5/1
  ERROR CONTROLLER VELOCITY/2(vd_ec) -> Sum6/2
  INTERNAL REFERENCE MODEL VELOCITY/4(u_ref) -> ERROR CONTROLLER VELOCITY/1(u_ref)
  [u_des] -> INTERNAL REFERENCE MODEL VELOCITY/1(u_cmd)
  [v_des] -> INTERNAL REFERENCE MODEL VELOCITY/2(v_cmd)
  [w_des] -> INTERNAL REFERENCE MODEL VELOCITY/3(w_cmd)
  [Phi_cmd] -> Scope12/1, INTERNAL REFERENCE MODEL ATTITUDE/1(phi_cmd)
  [Theta_cmd] -> [theta_cmd_1], Scope12/2, INTERNAL REFERENCE MODEL ATTITUDE/2(theta_cmd)
  [yaw_des] -> INTERNAL REFERENCE MODEL ATTITUDE/3(psi_cmd), Scope12/3
  Vector Concatenate/1 -> Scope1/1, [dv_inner]
  MATLAB Function/1(B_inner) -> Scope2/1, Display/1, Pseudoinverse/1
  Pseudoinverse/1 -> MatrixMultiply/1, Scope4/1
  MatrixMultiply/1 -> Scope3/1, Sum8/1  "du"
  [omega_1_1] -> Vector Concatenate1/1
  [omega_2_1] -> Vector Concatenate1/2
  [omega_3_1] -> Vector Concatenate1/3
  [omega_4_1] -> Vector Concatenate1/4
  Vector Concatenate1/1 -> Sum7/2
  Constant2/1 -> Sum7/1
  Sum7/1 -> Sum8/2  "u"
  Sum8/1 -> Scope/1, Demux/1
  Demux/1 -> Motor_1_omega_input/1
  Demux/2 -> Motor_2_omega_input/1
  Demux/3 -> Motor_3_omega_input/1
  Demux/4 -> Motor_4_omega_input/1
  Sum4/1 -> Vector Concatenate/1
  Sum11/1 -> Vector Concatenate/2
  Sum13/1 -> Vector Concatenate/3
  [dv_inner] -> MatrixMultiply/2
  [T_increment] -> Gain/1
  Sum12/1 -> Sum19/1  "wd"
  Sum6/1 -> Sum18/1  "vd"
  Sum5/1 -> Sum17/1  "ud"
  Vector Concatenate3/1 -> Scope7/1, [dv_outer]
  Sum19/1 -> Vector Concatenate3/3
  Sum18/1 -> Vector Concatenate3/2
  Sum17/1 -> Vector Concatenate3/1
  [AxAyAz_earth_1] -> Demux3/1
  Demux3/3 -> Sum19/2
  Demux3/2 -> Sum18/2
  Demux3/1 -> Sum17/2
  [K_m_1] -> MATLAB Function/4(K_m)
  [Izz_1] -> MATLAB Function/3(Izz)
  [Iyy_1] -> MATLAB Function/2(Iyy)
  [Ixx_1] -> MATLAB Function/1(Ixx)
  [omega_3_1] -> MATLAB Function/8(Omega_3)
  [omega_1_1] -> MATLAB Function/6(Omega_1)
  [omega_4_1] -> MATLAB Function/9(Omega_4)
  [K_t_1] -> MATLAB Function/5(K_t)
  [b_1] -> MATLAB Function/10(b)
  [l_1] -> MATLAB Function/11(l)
  [omega_2_1] -> MATLAB Function/7(Omega_2)
  Pseudoinverse1/1 -> Scope11/1, MatrixMultiply1/1
  Sum20/1 -> [Phi_cmd]
  Demux5/1 -> Sum20/1
  [Phi_1] -> MATLAB Function1/2(Phi)
  Demux5/2 -> Sum16/1
  MatrixMultiply1/1 -> Demux5/1  "du"
  Sum21/1 -> Sum16/2  "u"
  [Theta_1] -> Sum21/2
  [m_1] -> MATLAB Function1/5(m)
  [T_1] -> MATLAB Function1/1(T)
  [dv_outer] -> MatrixMultiply1/2
  Constant1/1 -> Sum21/1
  [Phi_1] -> Sum15/2
  Sum16/1 -> [Theta_cmd]
  [Psi_1] -> MATLAB Function1/4(Psi)
  [Theta_1] -> MATLAB Function1/3(Theta)
  Demux5/3 -> [T_increment]
  Sum15/1 -> Sum20/2  "u"
  MATLAB Function1/1(B_outer) -> Pseudoinverse1/1, Scope9/1, Display1/1
  Constant3/1 -> Sum15/1
  INTERNAL REFERENCE MODEL ATTITUDE/4(pd_ref) -> ERROR CONTROLLER ATTITUDE/1(pd_ref)
  INTERNAL REFERENCE MODEL ATTITUDE/5(qd_ref) -> ERROR CONTROLLER ATTITUDE/2(qd_ref)
  INTERNAL REFERENCE MODEL ATTITUDE/6(rd_ref) -> ERROR CONTROLLER ATTITUDE/3(rd_ref)
  INTERNAL REFERENCE MODEL ATTITUDE/7(p_ref) -> ERROR CONTROLLER ATTITUDE/4(p_ref)
  INTERNAL REFERENCE MODEL ATTITUDE/8(q_ref) -> ERROR CONTROLLER ATTITUDE/5(q_ref)
  INTERNAL REFERENCE MODEL ATTITUDE/9(r_ref) -> ERROR CONTROLLER ATTITUDE/6(r_ref)
  INTERNAL REFERENCE MODEL ATTITUDE/10(phi_ref) -> ERROR CONTROLLER ATTITUDE/7(phi_ref)
  INTERNAL REFERENCE MODEL ATTITUDE/11(theta_ref) -> [theta_ref_1], ERROR CONTROLLER ATTITUDE/8(theta_ref)
  INTERNAL REFERENCE MODEL ATTITUDE/12(psi_ref) -> ERROR CONTROLLER ATTITUDE/9(psi_ref)
  INTERNAL REFERENCE MODEL ATTITUDE/1(pdd_ref) -> Sum4/1
  INTERNAL REFERENCE MODEL ATTITUDE/2(qdd_ref) -> Sum11/1
  INTERNAL REFERENCE MODEL ATTITUDE/3(rdd_ref) -> Sum13/1
  ERROR CONTROLLER ATTITUDE/1(pdd_ec) -> Sum4/2
  ERROR CONTROLLER ATTITUDE/2(qdd_ec) -> Sum11/2, [qdd_ec_1]
  ERROR CONTROLLER ATTITUDE/3(rdd_ec) -> Sum13/2
  Constant/1 -> MATLAB Function/12(K_act_inner)
  Gain/1 -> Vector Concatenate/4

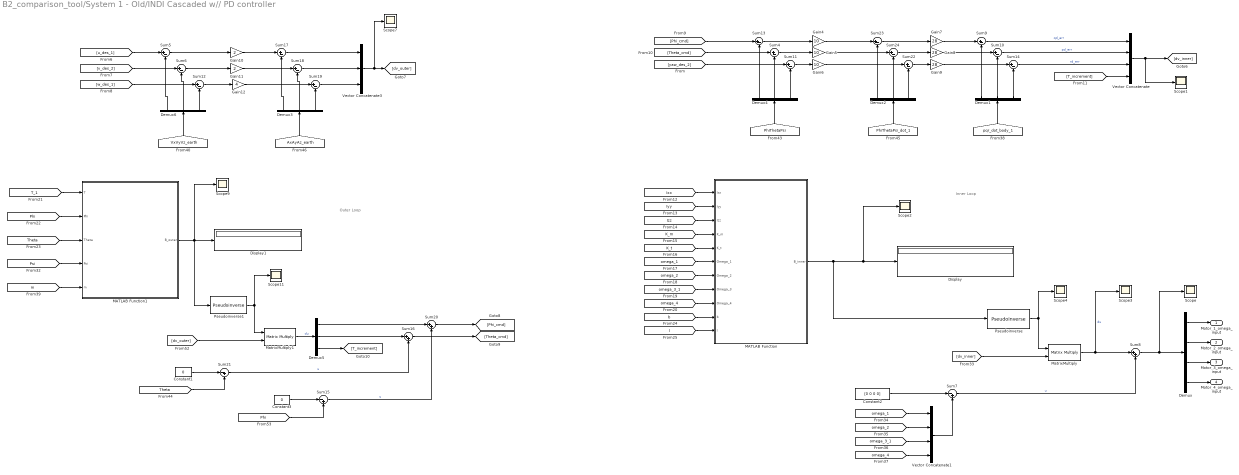
== system B2_comparison_tool/System 1 - Old/INDI Cascaded w// PD controller ==
  note: Inner Loop
  note: Outer Loop
  Constant1 : Constant  Value=0
  Constant2 : Constant  Value=[0 0 0 0]
  Constant3 : Constant  Value=0
  Demux : Demux
  Demux{1..6} (6 alike) : Demux  Outputs=3
  Display : Display
  Display1 : Display
  Gain10 : Gain  Gain=2
  Gain11 : Gain  Gain=2
  Gain12 : Gain  Gain=4
  Gain4 : Gain  Gain=10
  Gain5 : Gain  Gain=10
  Gain6 : Gain  Gain=10
  Gain7 : Gain  Gain=28
  Gain8 : Gain  Gain=28
  Gain9 : Gain  Gain=28
  MATLAB Function : MATLAB Function  TreatAsAtomicUnit=on
  MATLAB Function1 : MATLAB Function  TreatAsAtomicUnit=on
  MatrixMultiply : Product  Multiplication=Matrix(*)
  MatrixMultiply1 : Product  Multiplication=Matrix(*)
  Pseudoinverse : dspinverses/Pseudoinverse  wanterr=off  SimulateUsing=Interpreted execution
      settings: SourceProductBaseCode=DS
  Pseudoinverse1 : dspinverses/Pseudoinverse  wanterr=off  SimulateUsing=Interpreted execution
      settings: SourceProductBaseCode=DS
  Scope{,1..4,7,9,11} (8 alike) : Scope
  Sum{4..6,9..14,17..19,22..24} (15 alike) : Sum  Inputs=|+-
  Sum15 : Sum  Inputs=|-+
  Sum16 : Sum  Inputs=|++
  Sum20 : Sum  Inputs=|++
  Sum21 : Sum  Inputs=|-+
  Sum7 : Sum  Inputs=|-+
  Sum8 : Sum  Inputs=|++
  Vector Concatenate : Concatenate  NumInputs=4
  Vector Concatenate1 : Concatenate  NumInputs=4
  Vector Concatenate3 : Concatenate  NumInputs=3
  Motor_1_omega_input : Outport
  Motor_2_omega_input : Outport  Port=2
  Motor_3_omega_input : Outport  Port=3
  Motor_4_omega_input : Outport  Port=4
  wires:
  Vector Concatenate/1 -> Scope1/1, [dv_inner]
  [Ixx] -> MATLAB Function/1(Ixx)
  [Iyy] -> MATLAB Function/2(Iyy)
  [Izz] -> MATLAB Function/3(Izz)
  [K_m] -> MATLAB Function/4(K_m)
  [K_t] -> MATLAB Function/5(K_t)
  [omega_1] -> MATLAB Function/6(Omega_1)
  [omega_2] -> MATLAB Function/7(Omega_2)
  [omega_3_1] -> MATLAB Function/8(Omega_3)
  [omega_4] -> MATLAB Function/9(Omega_4)
  [b] -> MATLAB Function/10(b)
  [l] -> MATLAB Function/11(l)
  MATLAB Function/1(B_inner) -> Pseudoinverse/1, Scope2/1, Display/1
  Pseudoinverse/1 -> MatrixMultiply/1, Scope4/1
  MatrixMultiply/1 -> Scope3/1, Sum8/1  "du"
  [omega_1] -> Vector Concatenate1/1
  [omega_2] -> Vector Concatenate1/2
  [omega_3_1] -> Vector Concatenate1/3
  [omega_4] -> Vector Concatenate1/4
  Vector Concatenate1/1 -> Sum7/2
  Constant2/1 -> Sum7/1
  Sum7/1 -> Sum8/2  "u"
  Sum8/1 -> Scope/1, Demux/1
  Demux/1 -> Motor_1_omega_input/1
  Demux/2 -> Motor_2_omega_input/1
  Demux/3 -> Motor_3_omega_input/1
  Demux/4 -> Motor_4_omega_input/1
  Sum9/1 -> Vector Concatenate/1  "qd_err"
  Sum10/1 -> Vector Concatenate/2  "pd_err"
  Sum14/1 -> Vector Concatenate/3  "rd_err"
  [pqr_dot_body_1] -> Demux1/1
  Demux1/3 -> Sum14/2
  Demux1/2 -> Sum10/2
  Demux1/1 -> Sum9/2
  [dv_inner] -> MatrixMultiply/2
  [T_increment] -> Vector Concatenate/4
  [dv_outer] -> MatrixMultiply1/2
  Constant3/1 -> Sum15/1
  MATLAB Function1/1(B_outer) -> Pseudoinverse1/1, Scope9/1, Display1/1
  Sum15/1 -> Sum20/2  "u"
  Pseudoinverse1/1 -> Scope11/1, MatrixMultiply1/1
  [T_1] -> MATLAB Function1/1(T)
  [Phi] -> MATLAB Function1/2(Phi)
  [Theta] -> MATLAB Function1/3(Theta)
  [Psi] -> MATLAB Function1/4(Psi)
  [m] -> MATLAB Function1/5(m)
  Vector Concatenate3/1 -> [dv_outer], Scope7/1
  Sum19/1 -> Vector Concatenate3/3
  Sum18/1 -> Vector Concatenate3/2
  Sum17/1 -> Vector Concatenate3/1
  [AxAyAz_earth] -> Demux3/1
  Demux3/3 -> Sum19/2
  Demux3/2 -> Sum18/2
  Demux3/1 -> Sum17/2
  [PhiThetaPsi] -> Demux4/1
  Demux4/2 -> Sum4/2
  Demux4/1 -> Sum13/2
  Demux4/3 -> Sum11/2
  [yaw_des_2] -> Sum11/1
  [Theta_cmd] -> Sum4/1
  [Phi_cmd] -> Sum13/1
  Sum11/1 -> Gain6/1
  Sum4/1 -> Gain5/1
  Sum13/1 -> Gain4/1
  MatrixMultiply1/1 -> Demux5/1  "du"
  Demux5/3 -> [T_increment]
  Demux5/2 -> Sum16/1
  Demux5/1 -> Sum20/1
  [Phi] -> Sum15/2
  Constant1/1 -> Sum21/1
  [Theta] -> Sum21/2
  Sum21/1 -> Sum16/2  "u"
  Sum20/1 -> [Phi_cmd]
  Sum16/1 -> [Theta_cmd]
  Gain4/1 -> Sum23/1
  Gain5/1 -> Sum24/1
  Demux2/3 -> Sum22/2
  Demux2/1 -> Sum23/2
  Gain6/1 -> Sum22/1
  Demux2/2 -> Sum24/2
  Sum23/1 -> Gain7/1
  Sum24/1 -> Gain8/1
  [PhiThetaPsi_dot_1] -> Demux2/1
  Sum22/1 -> Gain9/1
  Gain7/1 -> Sum9/1
  Gain8/1 -> Sum10/1
  Gain9/1 -> Sum14/1
  Demux6/1 -> Sum5/2
  Sum5/1 -> Gain10/1
  [VxVyVz_earth] -> Demux6/1
  Demux6/2 -> Sum6/2
  Demux6/3 -> Sum12/2
  Sum6/1 -> Gain11/1
  Sum12/1 -> Gain12/1
  Gain10/1 -> Sum17/1
  Gain11/1 -> Sum18/1
  Gain12/1 -> Sum19/1
  [u_des_1] -> Sum5/1
  [v_des_2] -> Sum6/1
  [w_des_1] -> Sum12/1

== system B2_comparison_tool/System 1 - Old/INDI w// RSPI ==
  " " : Constant  Value=[0;0;0;0]
  Constant : Constant  Value=0
  Constant1 : Constant  Value=max_omega_motor
  Constant2 : Constant  Value=max_motor_rate
  Constant3 : Constant  Value=sampling_time
  Constant4 : Constant  Value=2
  Constant5 : Constant  Value=0
  Demux : Demux
  Demux1 : Demux  Outputs=3
  Demux2 : Demux  Outputs=3
  ERROR CONTROLLER ATTITUDE : Subsystem
  ERROR CONTROLLER VELOCITY : Subsystem
  INTERNAL REFERENCE MODEL ATTITUDE : Subsystem
  INTERNAL REFERENCE MODEL VELOCITY : Subsystem
  MATLAB Function : MATLAB Function  TreatAsAtomicUnit=on
  Scope : Scope
  Scope1 : Scope
  Scope5 : Scope  NumInputPorts=3
  Scope6 : Scope  NumInputPorts=3
  Sum{9..10,14..17} (6 alike) : Sum  Inputs=|+-
  Sum{4..6,11..13} (6 alike) : Sum  Inputs=|++
  Vector Concatenate : Concatenate  NumInputs=6
  pqr_ref : Scope  NumInputPorts=3
  uvw_ref : Scope  NumInputPorts=3
  Motor_1_omega_input : Outport
  Motor_2_omega_input : Outport  Port=2
  Motor_3_omega_input : Outport  Port=3
  Motor_4_omega_input : Outport  Port=4
  wires:
  [Ixx] -> MATLAB Function/1(Ixx)
  [Iyy] -> MATLAB Function/2(Iyy)
  [Izz] -> MATLAB Function/3(Izz)
  [K_m] -> MATLAB Function/4(K_m)
  [K_t] -> MATLAB Function/5(K_t)
  [omega_1] -> MATLAB Function/6(Omega_1)
  [omega_2] -> MATLAB Function/7(Omega_2)
  [omega_3_1] -> MATLAB Function/8(Omega_3)
  [omega_4] -> MATLAB Function/9(Omega_4)
  [Phi] -> MATLAB Function/10(Phi)
  [Psi] -> MATLAB Function/11(Psi)
  [Theta] -> MATLAB Function/12(Theta)
  [m] -> MATLAB Function/15(m)
  Demux/1 -> Motor_1_omega_input/1
  Demux/2 -> Motor_2_omega_input/1
  Demux/3 -> Motor_3_omega_input/1
  Demux/4 -> Motor_4_omega_input/1
  [dv] -> MATLAB Function/16(dv)
  " "/1 -> MATLAB Function/17(desired_u)
  Constant1/1 -> MATLAB Function/18(max_omega_motor)
  Constant2/1 -> MATLAB Function/19(max_motor_rate)
  Constant3/1 -> MATLAB Function/20(sampling_time)
  MATLAB Function/1(u_out) -> Scope/1, Demux/1
  Constant4/1 -> MATLAB Function/21(max_iter)
  Constant/1 -> INTERNAL REFERENCE MODEL ATTITUDE/1(phi_cmd)
  Constant5/1 -> INTERNAL REFERENCE MODEL ATTITUDE/2(theta_cmd)
  INTERNAL REFERENCE MODEL VELOCITY/5(v_ref) -> ERROR CONTROLLER VELOCITY/2(v_ref), uvw_ref/2
  INTERNAL REFERENCE MODEL ATTITUDE/6(r_ref) -> ERROR CONTROLLER ATTITUDE/3(r_ref), pqr_ref/3
  Demux1/3 -> Sum14/2
  [u_des_1] -> INTERNAL REFERENCE MODEL VELOCITY/1(u_cmd)
  Sum9/1 -> Vector Concatenate/1
  ERROR CONTROLLER VELOCITY/1(ud_ec) -> Scope6/1, Sum5/2
  [yaw_des_2] -> INTERNAL REFERENCE MODEL ATTITUDE/3(psi_cmd)
  Vector Concatenate/1 -> Scope1/1, [dv]
  INTERNAL REFERENCE MODEL ATTITUDE/3(rd_ref) -> Sum13/1
  Demux1/1 -> Sum9/2
  INTERNAL REFERENCE MODEL ATTITUDE/5(q_ref) -> ERROR CONTROLLER ATTITUDE/2(q_ref), pqr_ref/2
  Demux2/3 -> Sum17/2
  Sum16/1 -> Vector Concatenate/5
  [pqr_dot_body_1] -> Demux1/1
  [AxAyAz_earth] -> Demux2/1
  Sum12/1 -> Sum17/1
  Sum10/1 -> Vector Concatenate/2
  Sum14/1 -> Vector Concatenate/3
  ERROR CONTROLLER ATTITUDE/2(qd_ec) -> Scope5/2, Sum11/2
  Demux2/2 -> Sum16/2
  ERROR CONTROLLER ATTITUDE/1(pd_ec) -> Scope5/1, Sum4/2
  Sum15/1 -> Vector Concatenate/4
  Sum17/1 -> Vector Concatenate/6
  ERROR CONTROLLER VELOCITY/3(wd_ec) -> Scope6/3, Sum12/2
  Sum11/1 -> Sum10/1
  INTERNAL REFERENCE MODEL VELOCITY/4(u_ref) -> uvw_ref/1, ERROR CONTROLLER VELOCITY/1(u_ref)
  Sum13/1 -> Sum14/1
  Sum6/1 -> Sum16/1
  INTERNAL REFERENCE MODEL VELOCITY/6(w_ref) -> ERROR CONTROLLER VELOCITY/3(w_ref), uvw_ref/3
  [v_des_2] -> INTERNAL REFERENCE MODEL VELOCITY/2(v_cmd)
  Demux1/2 -> Sum10/2
  ERROR CONTROLLER VELOCITY/2(vd_ec) -> Scope6/2, Sum6/2
  INTERNAL REFERENCE MODEL VELOCITY/1(ud_ref) -> Sum5/1
  [w_des_1] -> INTERNAL REFERENCE MODEL VELOCITY/3(w_cmd)
  Sum5/1 -> Sum15/1
  INTERNAL REFERENCE MODEL VELOCITY/3(wd_ref) -> Sum12/1
  Demux2/1 -> Sum15/2
  INTERNAL REFERENCE MODEL ATTITUDE/7(phi_ref) -> ERROR CONTROLLER ATTITUDE/4(phi_ref)
  INTERNAL REFERENCE MODEL ATTITUDE/8(theta_ref) -> ERROR CONTROLLER ATTITUDE/5(theta_ref)
  INTERNAL REFERENCE MODEL ATTITUDE/1(pd_ref) -> Sum4/1
  INTERNAL REFERENCE MODEL VELOCITY/2(vd_ref) -> Sum6/1
  Sum4/1 -> Sum9/1
  INTERNAL REFERENCE MODEL ATTITUDE/4(p_ref) -> pqr_ref/1, ERROR CONTROLLER ATTITUDE/1(p_ref)
  INTERNAL REFERENCE MODEL ATTITUDE/9(psi_ref) -> ERROR CONTROLLER ATTITUDE/6(psi_ref)
  INTERNAL REFERENCE MODEL ATTITUDE/2(qd_ref) -> Sum11/1
  ERROR CONTROLLER ATTITUDE/3(qr_ec) -> Scope5/3, Sum13/2
  [b] -> MATLAB Function/13(b)
  [l] -> MATLAB Function/14(l)

== system B2_comparison_tool/System 1 - Old/Quadcopter Characteristics ==
  Gravity : Constant  Value=9.80665
  Moment Gain : Constant  Value=6.68*10^-10
  Plate Distance from CG : Constant  Value=0.1
  Plate Radius (cm) : Constant  Value=0.30
  Quad Inertia Ixx [kg*m^2] : Constant  Value=0.0012458
  Quad Inertia Iyy [kg*m^2] : Constant  Value=0.001500
  Quad Inertia Izz [kg*m^2] : Constant  Value=0.0001500
  Quad Mass [kg] : Constant  Value=0.4
  Thrust Gain : Constant  Value=6.557*10^-8
  lx1 : Constant  Value=0.095
  lx2 : Constant  Value=0.08
  tag scope: Ixx_1=global, Iyy_1=global, Izz_1=global, K_m_1=global, K_t_1=global, b_1=global, g_1=global, l_1=global, l_plate_1=global, m_1=global, r_plate_1=global
  wires:
  Quad Inertia Ixx [kg*m^2]/1 -> [Ixx_1]
  Quad Inertia Iyy [kg*m^2]/1 -> [Iyy_1]
  Quad Inertia Izz [kg*m^2]/1 -> [Izz_1]
  Quad Mass [kg]/1 -> [m_1]
  Thrust Gain/1 -> [K_t_1]
  Moment Gain/1 -> [K_m_1]
  lx1/1 -> [b_1]
  lx2/1 -> [l_1]
  Plate Radius (cm)/1 -> [r_plate_1]
  Plate Distance from CG/1 -> [l_plate_1]
  Gravity/1 -> [g_1]

== system B2_comparison_tool/System 0 - New/Equations of Motion/Vehicle Dynamics ==
  note: Attitude Calculations
  note: Rotation Matrices Calculations
  note: Position Calculations
  Ixx : Inport
  Iyy : Inport  Port=2
  Izz : Inport  Port=3
  mass : Inport  Port=4
  Force in earth frame : Inport  Port=5
  Moments in the body frame : Inport  Port=6
  Demux : Demux  Outputs=3
  Demux2 : Demux  Outputs=3
  Disturbance Block : Subsystem
  Divide : Product  Inputs=*/
  Divide1 : Product  Inputs=*/
  Inertia Iij : Constant  Value=0
  Integrator{1..3,12} (4 alike) : Integrator
  Invert 3x3 Matrix : aerolibutil/Invert  3x3 Matrix
  Matrix Multiply{,1..4} (5 alike) : Product  Multiplication=Matrix(*)
  Omega_I_Omega : Subsystem
  Scope : Scope  NumInputPorts=3
  Subtract : Sum
  Subtract1 : Sum  Inputs=-+
  Sum : Sum  Inputs=|++
  Sum1 : Sum  Inputs=|++
  Sum2 : Sum  Inputs=|++
  Symmetric Inertia Tensor : aerolibbdyn/Symmetric Inertia Tensor
      settings: SourceProductBaseCode=AE
  Transpose : Math  Operator=transpose  SaturateOnIntegerOverflow=on
  Vector Concatenate : Concatenate  NumInputs=3
  Vector Concatenate1 : Concatenate  NumInputs=3
  body_to_ground_transorm : MATLAB Function  Description=|  TreatAsAtomicUnit=on
      | This function computes the rotational matrix to pass from the body frame to the world frame. 
      | Takes as inpout the euler angles.
  euler_rates_to_pqr : MATLAB Function  TreatAsAtomicUnit=on
  g1 : Constant  Value=9.81  VectorParams1D=off
  k : Constant  Value=0  VectorParams1D=off
  pqr_to_euler_rates : MATLAB Function  TreatAsAtomicUnit=on
  pqr_dot_body : Outport
  PhiThetaPsi_dot : Outport  Port=2
  PhiThetaPsi : Outport  Port=3
  R : Outport  Port=4
  T : Outport  Port=5
  R_bg : Outport  Port=6
  AxAyAz_earth : Outport  Port=7
  VxVyVz_earth : Outport  Port=8
  xyz_earth : Outport  Port=9
  AxAyAz_body : Outport  Port=10
  VxVyVz_body : Outport  Port=11
  xyz_body : Outport  Port=12
  wires:
  Transpose/1 -> Matrix Multiply1/1, Matrix Multiply2/1, Matrix Multiply4/1
  Matrix Multiply2/1 -> VxVyVz_body/1
  Matrix Multiply1/1 -> xyz_body/1
  Subtract/1 -> Integrator2/1, Matrix Multiply4/2, AxAyAz_earth/1  "AxAyAz_earth"
  Matrix Multiply4/1 -> AxAyAz_body/1
  body_to_ground_transorm/1(R_bg) -> Transpose/1, R_bg/1
  Integrator2/1 -> Matrix Multiply2/2, VxVyVz_earth/1, Integrator3/1  "VxVyVz_earth"
  Force in earth frame/1 -> Divide/1
  Demux2/3 -> body_to_ground_transorm/3(Psi)  "Psi"
  Demux2/2 -> euler_rates_to_pqr/2(Theta), body_to_ground_transorm/2(Theta), pqr_to_euler_rates/2(Theta)  "Theta"
  euler_rates_to_pqr/1(R) -> R/1
  pqr_to_euler_rates/1(T) -> Matrix Multiply3/1, T/1
  Matrix Multiply/1 -> Demux/1
  Integrator12/1 -> Matrix Multiply3/2, Omega_I_Omega/1(pqr_body)  "pqr_body"
  Integrator3/1 -> Matrix Multiply1/2, xyz_earth/1  "xyz_earth"
  Ixx/1 -> Symmetric Inertia Tensor/1
  k/1 -> Vector Concatenate/2, Vector Concatenate/1
  Vector Concatenate/1 -> Subtract/1
  Integrator1/1 -> PhiThetaPsi/1, Demux2/1  "Euler_angles"
  g1/1 -> Vector Concatenate/3
  Moments in the body frame/1 -> Subtract1/2
  Demux2/1 -> euler_rates_to_pqr/1(Phi), pqr_to_euler_rates/1(Phi), body_to_ground_transorm/1(Phi)  "Phi"
  Vector Concatenate1/1 -> Integrator12/1, pqr_dot_body/1
  Matrix Multiply3/1 -> PhiThetaPsi_dot/1, Integrator1/1  "Euler_rates"
  mass/1 -> Divide/2
  Omega_I_Omega/1(Final product) -> Subtract1/1
  Subtract1/1 -> Matrix Multiply/2
  Invert 3x3 Matrix/1 -> Matrix Multiply/1
  Inertia Iij/1 -> Symmetric Inertia Tensor/5, Symmetric Inertia Tensor/3, Symmetric Inertia Tensor/2
  Divide/1 -> Subtract/2
  Symmetric Inertia Tensor/1 -> Invert 3x3 Matrix/1, Omega_I_Omega/2(Inertia)
  Iyy/1 -> Symmetric Inertia Tensor/4
  Izz/1 -> Symmetric Inertia Tensor/6
  [Fz_earth] -> Divide1/1
  [m] -> Divide1/2
  Divide1/1 -> Scope/1
  [Az_earth] -> Scope/2
  [g] -> Scope/3
  Demux/1 -> Sum/1
  Sum/1 -> Vector Concatenate1/1
  Sum2/1 -> Vector Concatenate1/3
  Sum1/1 -> Vector Concatenate1/2
  Demux/2 -> Sum1/1
  Demux/3 -> Sum2/1
  Disturbance Block/1(Total Disturbance) -> ?

== system B2_comparison_tool/System 0 - New/Force and Moment Calculation/Forces and Moments due to Aerodynamic Forces ==
  z_earth : Inport
  R_bg : Inport  Port=2
  Aerodynamic Forces Calculator : MATLAB Function  TreatAsAtomicUnit=on
  Constant : Constant  Value=0
  Gain : Gain  Gain=-1
  ISA Atmosphere Model : aerolibatmos2/ISA Atmosphere Model  custom=off  g=9.80665  gamma=1.4  R=287.0531  L=0.0065  h_trop=11000  h_strat=20000  rho0=1.225  P0=101325  T0=288.15  h0=0
  Matrix Multiply1 : Product  Multiplication=Matrix(*)
  Radians to Degrees : simulink_extras/Transformations/Radians to Degrees
  Radians to Degrees1 : simulink_extras/Transformations/Radians to Degrees
  Scope : Scope  NumInputPorts=6
  Scope1 : Scope  NumInputPorts=2
  Scope2 : Scope  NumInputPorts=2
  Scope3 : Scope  NumInputPorts=2
  Scope4 : Scope
  Switch : Switch  Criteria=u2 > Threshold
  Terminator : Terminator
  Terminator1 : Terminator
  Terminator2 : Terminator
  Vector Concatenate : Concatenate  NumInputs=3
  Vector Concatenate1 : Concatenate  NumInputs=3
  F_aero : Outport
  M_aero : Outport  Port=2
  tag scope: alpha=global, beta=global, rho=global
  wires:
  ISA Atmosphere Model/2 -> Terminator1/1
  ISA Atmosphere Model/1 -> Terminator/1
  ISA Atmosphere Model/3 -> Terminator2/1
  z_earth/1 -> Gain/1
  ISA Atmosphere Model/4 -> Scope4/1, [rho]
  Aerodynamic Forces Calculator/3(Fz_body) -> Scope/3, Vector Concatenate/3  "Fz_body"
  Aerodynamic Forces Calculator/2(Fy_body) -> Scope/2, Vector Concatenate/2  "Fy_body"
  Matrix Multiply1/1 -> F_aero/1
  R_bg/1 -> Matrix Multiply1/1
  Aerodynamic Forces Calculator/1(Fx_body) -> Scope/1, Vector Concatenate/1  "Fx_body"
  Vector Concatenate/1 -> Matrix Multiply1/2
  Aerodynamic Forces Calculator/4(L_aero) -> Scope/4, Vector Concatenate1/1  "Mx"
  Aerodynamic Forces Calculator/5(M_aero) -> Scope/5, Vector Concatenate1/2  "My"
  Aerodynamic Forces Calculator/6(N_aero) -> Scope/6, Vector Concatenate1/3  "Mz"
  Vector Concatenate1/1 -> M_aero/1
  [Vx_body] -> Aerodynamic Forces Calculator/1(xd_body)
  [Vy_body] -> Aerodynamic Forces Calculator/2(yd_body)
  [Vz_body] -> Aerodynamic Forces Calculator/3(zd_body)
  [rho] -> Aerodynamic Forces Calculator/4(rho)
  [r_plate] -> Aerodynamic Forces Calculator/5(r_plate)
  [l_plate] -> Aerodynamic Forces Calculator/6(l_plate)
  Gain/1 -> Switch/2, Switch/1
  Constant/1 -> Switch/3
  Switch/1 -> ISA Atmosphere Model/1
  Aerodynamic Forces Calculator/7(Cl) -> Scope1/1  "Cl"
  Aerodynamic Forces Calculator/8(Cd) -> Scope1/2  "Cd"
  Aerodynamic Forces Calculator/9(L) -> Scope2/1  "L"
  Aerodynamic Forces Calculator/10(D) -> Scope2/2  "D"
  Aerodynamic Forces Calculator/11(alpha) -> [alpha], Radians to Degrees/1  "alpha"
  Aerodynamic Forces Calculator/12(beta) -> [beta], Radians to Degrees1/1  "beta"
  Radians to Degrees/1 -> Scope3/1
  Radians to Degrees1/1 -> Scope3/2

== system B2_comparison_tool/System 0 - New/INDI Block/ERROR CONTROLLER ATTITUDE ==
  p_ref : Inport
  q_ref : Inport  Port=2
  r_ref : Inport  Port=3
  phi_ref : Inport  Port=4
  theta_ref : Inport  Port=5
  psi_ref : Inport  Port=6
  Demux5 : Demux  Outputs=3
  Gain{,1..5} (6 alike) : Gain
  Sum{,1,3..4,6..7} (6 alike) : Sum  Inputs=|+-
  Sum2 : Sum  Inputs=|++
  Sum5 : Sum  Inputs=|++
  Sum8 : Sum  Inputs=|++
  pd_ec : Outport
  qd_ec : Outport  Port=2
  qr_ec : Outport  Port=3
  wires:
  p_ref/1 -> Sum/1
  phi_ref/1 -> Sum1/1
  Sum/1 -> Gain/1
  Sum1/1 -> Gain1/1
  Gain/1 -> Sum2/1
  Gain1/1 -> Sum2/2
  Sum2/1 -> pd_ec/1
  Gain2/1 -> Sum5/1
  Sum3/1 -> Gain2/1
  Gain3/1 -> Sum5/2
  theta_ref/1 -> Sum4/1
  q_ref/1 -> Sum3/1
  Sum5/1 -> qd_ec/1
  Sum4/1 -> Gain3/1
  Gain4/1 -> Sum8/1
  Sum6/1 -> Gain4/1
  Gain5/1 -> Sum8/2
  psi_ref/1 -> Sum7/1
  r_ref/1 -> Sum6/1
  Sum8/1 -> qr_ec/1
  Sum7/1 -> Gain5/1
  [Phi] -> Sum1/2
  [Theta] -> Sum4/2
  [Psi] -> Sum7/2
  Demux5/1 -> Sum/2
  Demux5/2 -> Sum3/2
  Demux5/3 -> Sum6/2
  [PhiThetaPsi_dot] -> Demux5/1
